simulink model "TideVCU"  (R2021b)
settings: Solver=FixedStepDiscrete  StartTime=0.0  StopTime=10.0  RelTol=1e-3
undefined symbols (not defined in the file): dataName, enumName, enumValue, GCM, raptor_get_safe_string
libraries: Raptor_lib x93, simulink x8
(part 2 of 3)

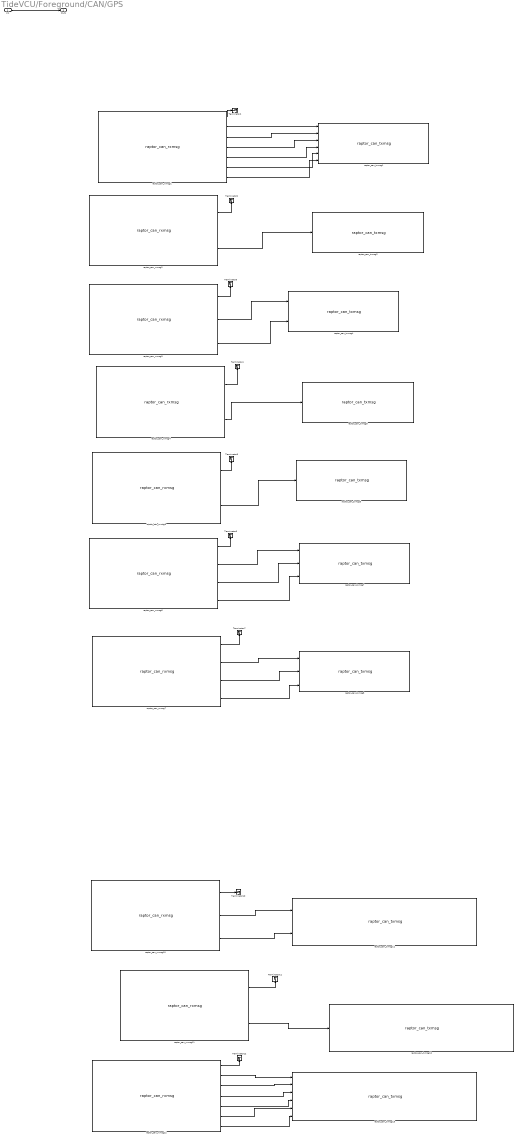
== system TideVCU/Foreground/CAN/GPS ==
  In1 : Inport
  Terminator{1..7,10..12} (10 alike) : Terminator
  raptor_can_rxmsg1 : Raptor_lib/CAN/raptor_can_rxmsg  canDefinition=struct('dbcFile', 'gps_out.dbc','message', 'accelxyz_temp_vertaxis_orientati','comment', '','signals', {{'accelx','accely','accelz','orientation','temp','vert_axis'}},'enabled', [ 1 1 1 1 1 1;],'scaled', [ 1 1 1 1 1 1;],'canBus', '''CAN1''','messageID', [ 1536;],'idMask', [ 536870911;],'payloadMask', [],'payloadValue', [],'period', [ 0;],'mailbox', '''''','queueSize', [ 1;],'label', [ 0;],'ver', [ 2;],'showID', [ 0;],'showRaw', [ 0;],'showRawMsg', [ 0;],'showAge', [ 1;],'fill', [ 0;],'editID', [ 0;],'signalOrder', [ 1;],'signalAscDes', [ 1;])  canBus='CAN1'  mailbox=''  payloadMask=[]  payloadValue=[]  idMask=hex2dec('1FFFFFFF')  queueSize=1  showID=0  label=0  fill=0  id=1536  showRaw=0  showAge=1  signalOrder=1  signalInfo={{struct('Name', 'accelx','Startbit', [ 0;],'SignalSize', [ 16;],'ByteOrder', 'LittleEndian','ValueType', 'SIGNED','Class', 'int16','Signed', [ 1;],'Factor', [ 3.91;],'Offset', [ 0;],'Min', [ 0;],'Max', [ 0;],'Units', '','Comment', '','StartBit', [ 0;]),struct('Name', 'accely','Startbit', [ 0;],'SignalSize', [ 16;],'ByteOrder', 'LittleEndian','ValueType', 'SIGNED','Class', 'int16','Signed', [ 1;],'Factor', [ 3.91;],'Offset', [ 0;],'Min', [ 0;],'Max', [ 0;],'Units', '','Comment', '','StartBit', [ 16;]),struct('Name', 'accelz','Startbit', [ 0;],'SignalSize', [ 16;],'ByteOrder', 'LittleEndian','ValueType', 'SIGNED','Class', 'int16','Signed', [ 1;],'Factor', [ 3.91;],'Offset', [ 0;],'Min', [ 0;],'Max', [ 0;],'Units', '','Comment', '','StartBit', [ 32;]),struct('Name', 'orientation','Startbit', [ 0;],'SignalSize', [ 3;],'ByteOrder', 'LittleEndian','ValueType', 'SIGNED','Class', 'int8','Signed', [ 1;],'Factor', [ 1;],'Offset', [ 0;],'Min', [ 0;],'Max', [ 0;],'Units', '','Comment', '','StartBit', [ 58;]),struct('Name', 'temp','Startbit', [ 0;],'SignalSize', [ 8;],'ByteOrder', 'LittleEndian','ValueType', 'SIGNED','Class', 'int8','Signed', [ 1;],'Factor', [ 0.5;],'Offset', [ 24;],'Min', [ 0;],'Max', [ 0;],'Units', 'c','Comment', '','StartBit', [ 48;]),struct('Name', 'vert_axis','Startbit', [ 0;],'SignalSize', [ 2;],'ByteOrder', 'LittleEndian','ValueType', 'SIGNED','Class', 'int8','Signed', [ 1;],'Factor', [ 1;],'Offset', [ 0;],'Min', [ 0;],'Max', [ 0;],'Units', '','Comment', '','StartBit', [ 56;])}}  showRawMsg=0
      settings: SourceProductName=Raptor
  raptor_can_rxmsg10 : Raptor_lib/CAN/raptor_can_rxmsg  canDefinition=struct('dbcFile', 'gps_out.dbc','message', 'rotation_xy','comment', '','signals', {{'rotationx','rotationy'}},'enabled', [ 1 1;],'scaled', [ 1 1;],'canBus', '''CAN2''','messageID', [ 1552;],'idMask', [ 536870911;],'payloadMask', [],'payloadValue', [],'period', [ 0;],'mailbox', '''''','queueSize', [ 1;],'label', [ 0;],'ver', [ 2;],'showID', [ 0;],'showRaw', [ 0;],'showRawMsg', [ 0;],'showAge', [ 1;],'fill', [ 0;],'editID', [ 0;],'signalOrder', [ 1;],'signalAscDes', [ 1;])  canBus='CAN2'  mailbox=''  payloadMask=[]  payloadValue=[]  idMask=hex2dec('1FFFFFFF')  queueSize=1  showID=0  label=0  fill=0  id=1552  showRaw=0  showAge=1  signalOrder=1  signalInfo={{struct('Name', 'rotationx','Startbit', [ 0;],'SignalSize', [ 32;],'ByteOrder', 'LittleEndian','ValueType', 'FLOAT32','Class', 'single','Signed', [ 1;],'Factor', [ 1;],'Offset', [ 0;],'Min', [ 0;],'Max', [ 0;],'Units', '','Comment', '','StartBit', [ 0;]),struct('Name', 'rotationy','Startbit', [ 0;],'SignalSize', [ 32;],'ByteOrder', 'LittleEndian','ValueType', 'FLOAT32','Class', 'single','Signed', [ 1;],'Factor', [ 1;],'Offset', [ 0;],'Min', [ 0;],'Max', [ 0;],'Units', '','Comment', '','StartBit', [ 32;])}}  showRawMsg=0
      settings: SourceProductName=Raptor
  raptor_can_rxmsg11 : Raptor_lib/CAN/raptor_can_rxmsg  canDefinition=struct('dbcFile', 'gps_out.dbc','message', 'rotationz','comment', '','signals', {{'rotationz'}},'enabled', [ 1;],'scaled', [ 1;],'canBus', '''CAN2''','messageID', [ 1553;],'idMask', [ 536870911;],'payloadMask', [],'payloadValue', [],'period', [ 0;],'mailbox', '''''','queueSize', [ 1;],'label', [ 0;],'ver', [ 2;],'showID', [ 0;],'showRaw', [ 0;],'showRawMsg', [ 0;],'showAge', [ 1;],'fill', [ 0;],'editID', [ 0;],'signalOrder', [ 1;],'signalAscDes', [ 1;])  canBus='CAN2'  mailbox=''  payloadMask=[]  payloadValue=[]  idMask=hex2dec('1FFFFFFF')  queueSize=1  showID=0  label=0  fill=0  id=1553  showRaw=0  showAge=1  signalOrder=1  signalInfo={{struct('Name', 'rotationz','Startbit', [ 0;],'SignalSize', [ 32;],'ByteOrder', 'LittleEndian','ValueType', 'FLOAT32','Class', 'single','Signed', [ 1;],'Factor', [ 1;],'Offset', [ 0;],'Min', [ 0;],'Max', [ 0;],'Units', '','Comment', '','StartBit', [ 0;])}}  showRawMsg=0
      settings: SourceProductName=Raptor
  raptor_can_rxmsg12 : Raptor_lib/CAN/raptor_can_rxmsg  canDefinition=struct('dbcFile', 'gps_out.dbc','message', 'IO','comment', '','signals', {{'Device_ID','Din1_status','Din2_status','Dout_status','GPS_powerStatus','SD_present'}},'enabled', [ 1 1 1 1 1 1;],'scaled', [ 1 1 1 1 1 1;],'canBus', '''CAN2''','messageID', [ 1584;],'idMask', [ 536870911;],'payloadMask', [],'payloadValue', [],'period', [ 0;],'mailbox', '''''','queueSize', [ 1;],'label', [ 0;],'ver', [ 2;],'showID', [ 0;],'showRaw', [ 0;],'showRawMsg', [ 0;],'showAge', [ 1;],'fill', [ 0;],'editID', [ 0;],'signalOrder', [ 1;],'signalAscDes', [ 1;])  canBus='CAN2'  mailbox=''  payloadMask=[]  payloadValue=[]  idMask=hex2dec('1FFFFFFF')  queueSize=1  showID=0  label=0  fill=0  id=1584  showRaw=0  showAge=1  signalOrder=1  signalInfo={{struct('Name', 'Din1_status','Startbit', [ 0;],'SignalSize', [ 1;],'ByteOrder', 'LittleEndian','ValueType', 'UNSIGNED','Class', 'uint8','Signed', [ 0;],'Factor', [ 1;],'Offset', [ 0;],'Min', [ 0;],'Max', [ 0;],'Units', '','Comment', '','StartBit', [ 0;]),struct('Name', 'Din2_status','Startbit', [ 0;],'SignalSize', [ 1;],'ByteOrder', 'LittleEndian','ValueType', 'UNSIGNED','Class', 'uint8','Signed', [ 0;],'Factor', [ 1;],'Offset', [ 0;],'Min', [ 0;],'Max', [ 0;],'Units', '','Comment', '','StartBit', [ 1;]),struct('Name', 'Dout_status','Startbit', [ 0;],'SignalSize', [ 1;],'ByteOrder', 'LittleEndian','ValueType', 'UNSIGNED','Class', 'uint8','Signed', [ 0;],'Factor', [ 1;],'Offset', [ 0;],'Min', [ 0;],'Max', [ 0;],'Units', '','Comment', '','StartBit', [ 2;]),struct('Name', 'SD_present','Startbit', [ 0;],'SignalSize', [ 1;],'ByteOrder', 'LittleEndian','ValueType', 'UNSIGNED','Class', 'uint8','Signed', [ 0;],'Factor', [ 1;],'Offset', [ 0;],'Min', [ 0;],'Max', [ 0;],'Units', '','Comment', '','StartBit', [ 3;]),struct('Name', 'GPS_powerStatus','Startbit', [ 0;],'SignalSize', [ 1;],'ByteOrder', 'LittleEndian','ValueType', 'UNSIGNED','Class', 'uint8','Signed', [ 0;],'Factor', [ 1;],'Offset', [ 0;],'Min', [ 0;],'Max', [ 0;],'Units', '','Comment', '','StartBit', [ 4;]),struct('Name', 'Device_ID','Startbit', [ 0;],'SignalSize', [ 3;],'ByteOrder', 'LittleEndian','ValueType', 'UNSIGNED','Class', 'uint8','Signed', [ 0;],'Factor', [ 1;],'Offset', [ 0;],'Min', [ 0;],'Max', [ 0;],'Units', '','Comment', '','StartBit', [ 5;])}}  showRawMsg=0
      settings: SourceProductName=Raptor
  raptor_can_rxmsg2 : Raptor_lib/CAN/raptor_can_rxmsg  canDefinition=struct('dbcFile', 'gps_out.dbc','message', 'gps_altitude','comment', '','signals', {{'altitude'}},'enabled', [ 1;],'scaled', [ 1;],'canBus', '''CAN1''','messageID', [ 1572;],'idMask', [ 536870911;],'payloadMask', [],'payloadValue', [],'period', [ 0;],'mailbox', '''''','queueSize', [ 1;],'label', [ 0;],'ver', [ 2;],'showID', [ 0;],'showRaw', [ 0;],'showRawMsg', [ 0;],'showAge', [ 1;],'fill', [ 0;],'editID', [ 0;],'signalOrder', [ 1;],'signalAscDes', [ 1;])  canBus='CAN1'  mailbox=''  payloadMask=[]  payloadValue=[]  idMask=hex2dec('1FFFFFFF')  queueSize=1  showID=0  label=0  fill=0  id=1572  showRaw=0  showAge=1  signalOrder=1  signalInfo={{struct('Name', 'altitude','Startbit', [ 0;],'SignalSize', [ 32;],'ByteOrder', 'LittleEndian','ValueType', 'FLOAT32','Class', 'single','Signed', [ 1;],'Factor', [ 1;],'Offset', [ 0;],'Min', [ 0;],'Max', [ 0;],'Units', '','Comment', '','StartBit', [ 0;])}}  showRawMsg=0
      settings: SourceProductName=Raptor
  raptor_can_rxmsg3 : Raptor_lib/CAN/raptor_can_rxmsg  canDefinition=struct('dbcFile', 'gps_out.dbc','message', 'gps_course_speed','comment', '','signals', {{'gps_course','gps_speed'}},'enabled', [ 1 1;],'scaled', [ 1 1;],'canBus', '''CAN2''','messageID', [ 1569;],'idMask', [ 536870911;],'payloadMask', [],'payloadValue', [],'period', [ 0;],'mailbox', '''''','queueSize', [ 1;],'label', [ 0;],'ver', [ 2;],'showID', [ 0;],'showRaw', [ 0;],'showRawMsg', [ 0;],'showAge', [ 1;],'fill', [ 0;],'editID', [ 0;],'signalOrder', [ 1;],'signalAscDes', [ 1;])  canBus='CAN2'  mailbox=''  payloadMask=[]  payloadValue=[]  idMask=hex2dec('1FFFFFFF')  queueSize=1  showID=0  label=0  fill=0  id=1569  showRaw=0  showAge=1  signalOrder=1  signalInfo={{struct('Name', 'gps_course','Startbit', [ 0;],'SignalSize', [ 32;],'ByteOrder', 'LittleEndian','ValueType', 'FLOAT32','Class', 'single','Signed', [ 1;],'Factor', [ 1;],'Offset', [ 0;],'Min', [ 0;],'Max', [ 0;],'Units', '','Comment', 'float, degrees','StartBit', [ 0;]),struct('Name', 'gps_speed','Startbit', [ 0;],'SignalSize', [ 32;],'ByteOrder', 'LittleEndian','ValueType', 'FLOAT32','Class', 'single','Signed', [ 1;],'Factor', [ 1;],'Offset', [ 0;],'Min', [ 0;],'Max', [ 0;],'Units', '','Comment', 'float, km/h','StartBit', [ 32;])}}  showRawMsg=0
      settings: SourceProductName=Raptor
  raptor_can_rxmsg4 : Raptor_lib/CAN/raptor_can_rxmsg  canDefinition=struct('dbcFile', 'gps_out.dbc','message', 'gps_delusionsA','comment', '','signals', {{'hdop','pdop'}},'enabled', [ 0 1;],'scaled', [ 1 1;],'canBus', '''CAN2''','messageID', [ 1573;],'idMask', [ 536870911;],'payloadMask', [],'payloadValue', [],'period', [ 0;],'mailbox', '''''','queueSize', [ 1;],'label', [ 0;],'ver', [ 2;],'showID', [ 0;],'showRaw', [ 0;],'showRawMsg', [ 0;],'showAge', [ 1;],'fill', [ 0;],'editID', [ 0;],'signalOrder', [ 1;],'signalAscDes', [ 1;])  canBus='CAN2'  mailbox=''  payloadMask=[]  payloadValue=[]  idMask=hex2dec('1FFFFFFF')  queueSize=1  showID=0  label=0  fill=0  id=1573  showRaw=0  showAge=1  signalOrder=1  signalInfo={{struct('Name', 'hdop','Startbit', [ 0;],'SignalSize', [ 32;],'ByteOrder', 'LittleEndian','ValueType', 'FLOAT32','Class', 'single','Signed', [ 1;],'Factor', [ 1;],'Offset', [ 0;],'Min', [ 0;],'Max', [ 0;],'Units', '','Comment', 'lower=better','StartBit', [ 32;]),struct('Name', 'pdop','Startbit', [ 0;],'SignalSize', [ 32;],'ByteOrder', 'LittleEndian','ValueType', 'FLOAT32','Class', 'single','Signed', [ 1;],'Factor', [ 1;],'Offset', [ 0;],'Min', [ 0;],'Max', [ 0;],'Units', '','Comment', 'lower=better','StartBit', [ 0;])}}  showRawMsg=0
      settings: SourceProductName=Raptor
  raptor_can_rxmsg5 : Raptor_lib/CAN/raptor_can_rxmsg  canDefinition=struct('dbcFile', 'gps_out.dbc','message', 'gps_delusionsB','comment', '','signals', {{'vdop'}},'enabled', [ 1;],'scaled', [ 1;],'canBus', '''CAN2''','messageID', [ 1574;],'idMask', [ 536870911;],'payloadMask', [],'payloadValue', [],'period', [ 0;],'mailbox', '''''','queueSize', [ 1;],'label', [ 0;],'ver', [ 2;],'showID', [ 0;],'showRaw', [ 0;],'showRawMsg', [ 0;],'showAge', [ 1;],'fill', [ 0;],'editID', [ 0;],'signalOrder', [ 1;],'signalAscDes', [ 1;])  canBus='CAN2'  mailbox=''  payloadMask=[]  payloadValue=[]  idMask=hex2dec('1FFFFFFF')  queueSize=1  showID=0  label=0  fill=0  id=1574  showRaw=0  showAge=1  signalOrder=1  signalInfo={{struct('Name', 'vdop','Startbit', [ 0;],'SignalSize', [ 32;],'ByteOrder', 'LittleEndian','ValueType', 'FLOAT32','Class', 'single','Signed', [ 1;],'Factor', [ 1;],'Offset', [ 0;],'Min', [ 0;],'Max', [ 0;],'Units', '','Comment', 'lower=better','StartBit', [ 0;])}}  showRawMsg=0
      settings: SourceProductName=Raptor
  raptor_can_rxmsg6 : Raptor_lib/CAN/raptor_can_rxmsg  canDefinition=struct('dbcFile', 'gps_out.dbc','message', 'gps_latitude','comment', '','signals', {{'indicator_north_south','latitude_degrees','latitude_minutes'}},'enabled', [ 1 1 1;],'scaled', [ 1 1 1;],'canBus', '''CAN2''','messageID', [ 1571;],'idMask', [ 536870911;],'payloadMask', [],'payloadValue', [],'period', [ 0;],'mailbox', '''''','queueSize', [ 1;],'label', [ 0;],'ver', [ 2;],'showID', [ 0;],'showRaw', [ 0;],'showRawMsg', [ 0;],'showAge', [ 1;],'fill', [ 0;],'editID', [ 0;],'signalOrder', [ 1;],'signalAscDes', [ 1;])  canBus='CAN2'  mailbox=''  payloadMask=[]  payloadValue=[]  idMask=hex2dec('1FFFFFFF')  queueSize=1  showID=0  label=0  fill=0  id=1571  showRaw=0  showAge=1  signalOrder=1  signalInfo={{struct('Name', 'latitude_minutes','Startbit', [ 0;],'SignalSize', [ 32;],'ByteOrder', 'LittleEndian','ValueType', 'FLOAT32','Class', 'single','Signed', [ 1;],'Factor', [ 1;],'Offset', [ 0;],'Min', [ 0;],'Max', [ 0;],'Units', '','Comment', 'float','StartBit', [ 0;]),struct('Name', 'latitude_degrees','Startbit', [ 0;],'SignalSize', [ 16;],'ByteOrder', 'LittleEndian','ValueType', 'SIGNED','Class', 'int16','Signed', [ 1;],'Factor', [ 1;],'Offset', [ 0;],'Min', [ 0;],'Max', [ 0;],'Units', '','Comment', '','StartBit', [ 32;]),struct('Name', 'indicator_north_south','Startbit', [ 0;],'SignalSize', [ 8;],'ByteOrder', 'LittleEndian','ValueType', 'SIGNED','Class', 'int8','Signed', [ 1;],'Factor', [ 1;],'Offset', [ 0;],'Min', [ 0;],'Max', [ 0;],'Units', '','Comment', '0=init','StartBit', [ 48;])}}  showRawMsg=0
      settings: SourceProductName=Raptor
  raptor_can_rxmsg7 : Raptor_lib/CAN/raptor_can_rxmsg  canDefinition=struct('dbcFile', 'gps_out.dbc','message', 'gps_longitude','comment', '','signals', {{'indicator_East_West','longitude_degrees','longitude_minutes'}},'enabled', [ 1 1 1;],'scaled', [ 1 1 1;],'canBus', '''CAN2''','messageID', [ 1570;],'idMask', [ 536870911;],'payloadMask', [],'payloadValue', [],'period', [ 0;],'mailbox', '''''','queueSize', [ 1;],'label', [ 0;],'ver', [ 2;],'showID', [ 0;],'showRaw', [ 0;],'showRawMsg', [ 0;],'showAge', [ 1;],'fill', [ 0;],'editID', [ 0;],'signalOrder', [ 1;],'signalAscDes', [ 1;])  canBus='CAN2'  mailbox=''  payloadMask=[]  payloadValue=[]  idMask=hex2dec('1FFFFFFF')  queueSize=1  showID=0  label=0  fill=0  id=1570  showRaw=0  showAge=1  signalOrder=1  signalInfo={{struct('Name', 'longitude_minutes','Startbit', [ 0;],'SignalSize', [ 32;],'ByteOrder', 'LittleEndian','ValueType', 'FLOAT32','Class', 'single','Signed', [ 1;],'Factor', [ 1;],'Offset', [ 0;],'Min', [ 0;],'Max', [ 0;],'Units', '','Comment', 'float','StartBit', [ 0;]),struct('Name', 'longitude_degrees','Startbit', [ 0;],'SignalSize', [ 16;],'ByteOrder', 'LittleEndian','ValueType', 'SIGNED','Class', 'int16','Signed', [ 1;],'Factor', [ 1;],'Offset', [ 0;],'Min', [ 0;],'Max', [ 0;],'Units', '','Comment', '','StartBit', [ 32;]),struct('Name', 'indicator_East_West','Startbit', [ 0;],'SignalSize', [ 8;],'ByteOrder', 'LittleEndian','ValueType', 'UNSIGNED','Class', 'uint8','Signed', [ 0;],'Factor', [ 1;],'Offset', [ 0;],'Min', [ 0;],'Max', [ 0;],'Units', '','Comment', '0=init','StartBit', [ 48;])}}  showRawMsg=0
      settings: SourceProductName=Raptor
  raptor_can_txmsg1 : Raptor_lib/CAN/raptor_can_txmsg  canDefinition=struct('dbcFile', 'gps_out.dbc','message', 'accelxyz_temp_vertaxis_orientati','comment', '','signals', {{'accelx','accely','accelz','orientation','temp','vert_axis'}},'enabled', [ 1 1 1 1 1 1;],'scaled', [ 1 1 1 1 1 1;],'canBus', '''CAN1''','messageID', [ 1536;],'idMask', [ 536870911;],'payloadMask', [],'payloadValue', [],'period', [ 0;],'mailbox', '','queueSize', [ 1;],'label', [ 0;],'ver', [ 2;],'showID', [ 0;],'showRaw', [ 0;],'showRawMsg', [ 0;],'fill', [ 0;],'editID', [ 0;],'signalOrder', [ 1;],'signalAscDes', [ 1;])  canBus='CAN1'  queueSize=1  payloadMask=[]  payloadValue=[]  period=0  showID=0  label=0  idMask=hex2dec('1FFFFFFF')  fill=0  id=1536  showRaw=0  signalOrder=1  signalInfo={{struct('Name', 'accelx','Startbit', [ 0;],'SignalSize', [ 16;],'ByteOrder', 'LittleEndian','ValueType', 'SIGNED','Class', 'int16','Signed', [ 1;],'Factor', [ 3.91;],'Offset', [ 0;],'Min', [ 0;],'Max', [ 0;],'Units', '','Comment', '','StartBit', [ 0;]),struct('Name', 'accely','Startbit', [ 0;],'SignalSize', [ 16;],'ByteOrder', 'LittleEndian','ValueType', 'SIGNED','Class', 'int16','Signed', [ 1;],'Factor', [ 3.91;],'Offset', [ 0;],'Min', [ 0;],'Max', [ 0;],'Units', '','Comment', '','StartBit', [ 16;]),struct('Name', 'accelz','Startbit', [ 0;],'SignalSize', [ 16;],'ByteOrder', 'LittleEndian','ValueType', 'SIGNED','Class', 'int16','Signed', [ 1;],'Factor', [ 3.91;],'Offset', [ 0;],'Min', [ 0;],'Max', [ 0;],'Units', '','Comment', '','StartBit', [ 32;]),struct('Name', 'temp','Startbit', [ 0;],'SignalSize', [ 8;],'ByteOrder', 'LittleEndian','ValueType', 'SIGNED','Class', 'int8','Signed', [ 1;],'Factor', [ 0.5;],'Offset', [ 24;],'Min', [ 0;],'Max', [ 0;],'Units', 'c','Comment', '','StartBit', [ 48;]),struct('Name', 'vert_axis','Startbit', [ 0;],'SignalSize', [ 2;],'ByteOrder', 'LittleEndian','ValueType', 'SIGNED','Class', 'int8','Signed', [ 1;],'Factor', [ 1;],'Offset', [ 0;],'Min', [ 0;],'Max', [ 0;],'Units', '','Comment', '','StartBit', [ 56;]),struct('Name', 'orientation','Startbit', [ 0;],'SignalSize', [ 3;],'ByteOrder', 'LittleEndian','ValueType', 'SIGNED','Class', 'int8','Signed', [ 1;],'Factor', [ 1;],'Offset', [ 0;],'Min', [ 0;],'Max', [ 0;],'Units', '','Comment', '','StartBit', [ 58;])}}
      settings: SourceProductName=Raptor
  raptor_can_txmsg11 : Raptor_lib/CAN/raptor_can_txmsg  canDefinition=struct('dbcFile', 'gps_out.dbc','message', 'rotation_xy','comment', '','signals', {{'rotationx','rotationy'}},'enabled', [ 1 1;],'scaled', [ 1 1;],'canBus', '''CAN1''','messageID', [ 1552;],'idMask', [ 536870911;],'payloadMask', [],'payloadValue', [],'period', [ 0;],'mailbox', '','queueSize', [ 1;],'label', [ 0;],'ver', [ 2;],'showID', [ 0;],'showRaw', [ 0;],'showRawMsg', [ 0;],'fill', [ 0;],'editID', [ 0;],'signalOrder', [ 1;],'signalAscDes', [ 1;])  canBus='CAN1'  queueSize=1  payloadMask=[]  payloadValue=[]  period=0  showID=0  label=0  idMask=hex2dec('1FFFFFFF')  fill=0  id=1552  showRaw=0  signalOrder=1  signalInfo={{struct('Name', 'rotationx','Startbit', [ 0;],'SignalSize', [ 32;],'ByteOrder', 'LittleEndian','ValueType', 'FLOAT32','Class', 'single','Signed', [ 1;],'Factor', [ 1;],'Offset', [ 0;],'Min', [ 0;],'Max', [ 0;],'Units', '','Comment', '','StartBit', [ 0;]),struct('Name', 'rotationy','Startbit', [ 0;],'SignalSize', [ 32;],'ByteOrder', 'LittleEndian','ValueType', 'FLOAT32','Class', 'single','Signed', [ 1;],'Factor', [ 1;],'Offset', [ 0;],'Min', [ 0;],'Max', [ 0;],'Units', '','Comment', '','StartBit', [ 32;])}}
      settings: SourceProductName=Raptor
  raptor_can_txmsg12 : Raptor_lib/CAN/raptor_can_txmsg  canDefinition=struct('dbcFile', 'gps_out.dbc','message', 'rotationz','comment', '','signals', {{'rotationz'}},'enabled', [ 1;],'scaled', [ 1;],'canBus', '''CAN1''','messageID', [ 1553;],'idMask', [ 536870911;],'payloadMask', [],'payloadValue', [],'period', [ 0;],'mailbox', '','queueSize', [ 1;],'label', [ 0;],'ver', [ 2;],'showID', [ 0;],'showRaw', [ 0;],'showRawMsg', [ 0;],'fill', [ 0;],'editID', [ 0;],'signalOrder', [ 1;],'signalAscDes', [ 1;])  canBus='CAN1'  queueSize=1  payloadMask=[]  payloadValue=[]  period=0  showID=0  label=0  idMask=hex2dec('1FFFFFFF')  fill=0  id=1553  showRaw=0  signalOrder=1  signalInfo={{struct('Name', 'rotationz','Startbit', [ 0;],'SignalSize', [ 32;],'ByteOrder', 'LittleEndian','ValueType', 'FLOAT32','Class', 'single','Signed', [ 1;],'Factor', [ 1;],'Offset', [ 0;],'Min', [ 0;],'Max', [ 0;],'Units', '','Comment', '','StartBit', [ 0;])}}
      settings: SourceProductName=Raptor
  raptor_can_txmsg13 : Raptor_lib/CAN/raptor_can_txmsg  canDefinition=struct('dbcFile', 'gps_out.dbc','message', 'IO','comment', '','signals', {{'Device_ID','Din1_status','Din2_status','Dout_status','GPS_powerStatus','SD_present'}},'enabled', [ 1 1 1 1 1 1;],'scaled', [ 1 1 1 1 1 1;],'canBus', '''CAN1''','messageID', [ 1584;],'idMask', [ 536870911;],'payloadMask', [],'payloadValue', [],'period', [ 0;],'mailbox', '','queueSize', [ 1;],'label', [ 0;],'ver', [ 2;],'showID', [ 0;],'showRaw', [ 0;],'showRawMsg', [ 0;],'fill', [ 0;],'editID', [ 0;],'signalOrder', [ 1;],'signalAscDes', [ 1;])  canBus='CAN1'  queueSize=1  payloadMask=[]  payloadValue=[]  period=0  showID=0  label=0  idMask=hex2dec('1FFFFFFF')  fill=0  id=1584  showRaw=0  signalOrder=1  signalInfo={{struct('Name', 'Din1_status','Startbit', [ 0;],'SignalSize', [ 1;],'ByteOrder', 'LittleEndian','ValueType', 'UNSIGNED','Class', 'uint8','Signed', [ 0;],'Factor', [ 1;],'Offset', [ 0;],'Min', [ 0;],'Max', [ 0;],'Units', '','Comment', '','StartBit', [ 0;]),struct('Name', 'Din2_status','Startbit', [ 0;],'SignalSize', [ 1;],'ByteOrder', 'LittleEndian','ValueType', 'UNSIGNED','Class', 'uint8','Signed', [ 0;],'Factor', [ 1;],'Offset', [ 0;],'Min', [ 0;],'Max', [ 0;],'Units', '','Comment', '','StartBit', [ 1;]),struct('Name', 'Dout_status','Startbit', [ 0;],'SignalSize', [ 1;],'ByteOrder', 'LittleEndian','ValueType', 'UNSIGNED','Class', 'uint8','Signed', [ 0;],'Factor', [ 1;],'Offset', [ 0;],'Min', [ 0;],'Max', [ 0;],'Units', '','Comment', '','StartBit', [ 2;]),struct('Name', 'SD_present','Startbit', [ 0;],'SignalSize', [ 1;],'ByteOrder', 'LittleEndian','ValueType', 'UNSIGNED','Class', 'uint8','Signed', [ 0;],'Factor', [ 1;],'Offset', [ 0;],'Min', [ 0;],'Max', [ 0;],'Units', '','Comment', '','StartBit', [ 3;]),struct('Name', 'GPS_powerStatus','Startbit', [ 0;],'SignalSize', [ 1;],'ByteOrder', 'LittleEndian','ValueType', 'UNSIGNED','Class', 'uint8','Signed', [ 0;],'Factor', [ 1;],'Offset', [ 0;],'Min', [ 0;],'Max', [ 0;],'Units', '','Comment', '','StartBit', [ 4;]),struct('Name', 'Device_ID','Startbit', [ 0;],'SignalSize', [ 3;],'ByteOrder', 'LittleEndian','ValueType', 'UNSIGNED','Class', 'uint8','Signed', [ 0;],'Factor', [ 1;],'Offset', [ 0;],'Min', [ 0;],'Max', [ 0;],'Units', '','Comment', '','StartBit', [ 5;])}}
      settings: SourceProductName=Raptor
  raptor_can_txmsg2 : Raptor_lib/CAN/raptor_can_txmsg  canDefinition=struct('dbcFile', 'gps_out.dbc','message', 'gps_altitude','comment', '','signals', {{'altitude'}},'enabled', [ 1;],'scaled', [ 1;],'canBus', '''CAN1''','messageID', [ 1572;],'idMask', [ 536870911;],'payloadMask', [],'payloadValue', [],'period', [ 0;],'mailbox', '','queueSize', [ 1;],'label', [ 0;],'ver', [ 2;],'showID', [ 0;],'showRaw', [ 0;],'showRawMsg', [ 0;],'fill', [ 0;],'editID', [ 0;],'signalOrder', [ 1;],'signalAscDes', [ 1;])  canBus='CAN1'  queueSize=1  payloadMask=[]  payloadValue=[]  period=0  showID=0  label=0  idMask=hex2dec('1FFFFFFF')  fill=0  id=1572  showRaw=0  signalOrder=1  signalInfo={{struct('Name', 'altitude','Startbit', [ 0;],'SignalSize', [ 32;],'ByteOrder', 'LittleEndian','ValueType', 'FLOAT32','Class', 'single','Signed', [ 1;],'Factor', [ 1;],'Offset', [ 0;],'Min', [ 0;],'Max', [ 0;],'Units', '','Comment', '','StartBit', [ 0;])}}
      settings: SourceProductName=Raptor
  raptor_can_txmsg4 : Raptor_lib/CAN/raptor_can_txmsg  canDefinition=struct('dbcFile', 'gps_out.dbc','message', 'gps_course_speed','comment', '','signals', {{'gps_course','gps_speed'}},'enabled', [ 1 1;],'scaled', [ 1 1;],'canBus', '''CAN1''','messageID', [ 1569;],'idMask', [ 536870911;],'payloadMask', [],'payloadValue', [],'period', [ 0;],'mailbox', '','queueSize', [ 1;],'label', [ 0;],'ver', [ 2;],'showID', [ 0;],'showRaw', [ 0;],'showRawMsg', [ 0;],'fill', [ 0;],'editID', [ 0;],'signalOrder', [ 1;],'signalAscDes', [ 1;])  canBus='CAN1'  queueSize=1  payloadMask=[]  payloadValue=[]  period=0  showID=0  label=0  idMask=hex2dec('1FFFFFFF')  fill=0  id=1569  showRaw=0  signalOrder=1  signalInfo={{struct('Name', 'gps_course','Startbit', [ 0;],'SignalSize', [ 32;],'ByteOrder', 'LittleEndian','ValueType', 'FLOAT32','Class', 'single','Signed', [ 1;],'Factor', [ 1;],'Offset', [ 0;],'Min', [ 0;],'Max', [ 0;],'Units', '','Comment', 'float, degrees','StartBit', [ 0;]),struct('Name', 'gps_speed','Startbit', [ 0;],'SignalSize', [ 32;],'ByteOrder', 'LittleEndian','ValueType', 'FLOAT32','Class', 'single','Signed', [ 1;],'Factor', [ 1;],'Offset', [ 0;],'Min', [ 0;],'Max', [ 0;],'Units', '','Comment', 'float, km/h','StartBit', [ 32;])}}
      settings: SourceProductName=Raptor
  raptor_can_txmsg5 : Raptor_lib/CAN/raptor_can_txmsg  canDefinition=struct('dbcFile', 'gps_out.dbc','message', 'gps_delusionsA','comment', '','signals', {{'hdop','pdop'}},'enabled', [ 0 1;],'scaled', [ 1 1;],'canBus', '''CAN1''','messageID', [ 1573;],'idMask', [ 536870911;],'payloadMask', [],'payloadValue', [],'period', [ 0;],'mailbox', '','queueSize', [ 1;],'label', [ 0;],'ver', [ 2;],'showID', [ 0;],'showRaw', [ 0;],'showRawMsg', [ 0;],'fill', [ 0;],'editID', [ 0;],'signalOrder', [ 1;],'signalAscDes', [ 1;])  canBus='CAN1'  queueSize=1  payloadMask=[]  payloadValue=[]  period=0  showID=0  label=0  idMask=hex2dec('1FFFFFFF')  fill=0  id=1573  showRaw=0  signalOrder=1  signalInfo={{struct('Name', 'hdop','Startbit', [ 0;],'SignalSize', [ 32;],'ByteOrder', 'LittleEndian','ValueType', 'FLOAT32','Class', 'single','Signed', [ 1;],'Factor', [ 1;],'Offset', [ 0;],'Min', [ 0;],'Max', [ 0;],'Units', '','Comment', 'lower=better','StartBit', [ 32;]),struct('Name', 'pdop','Startbit', [ 0;],'SignalSize', [ 32;],'ByteOrder', 'LittleEndian','ValueType', 'FLOAT32','Class', 'single','Signed', [ 1;],'Factor', [ 1;],'Offset', [ 0;],'Min', [ 0;],'Max', [ 0;],'Units', '','Comment', 'lower=better','StartBit', [ 0;])}}
      settings: SourceProductName=Raptor
  raptor_can_txmsg6 : Raptor_lib/CAN/raptor_can_txmsg  canDefinition=struct('dbcFile', 'gps_out.dbc','message', 'gps_delusionsB','comment', '','signals', {{'vdop'}},'enabled', [ 1;],'scaled', [ 1;],'canBus', '''CAN1''','messageID', [ 1574;],'idMask', [ 536870911;],'payloadMask', [],'payloadValue', [],'period', [ 0;],'mailbox', '','queueSize', [ 1;],'label', [ 0;],'ver', [ 2;],'showID', [ 0;],'showRaw', [ 0;],'showRawMsg', [ 0;],'fill', [ 0;],'editID', [ 0;],'signalOrder', [ 1;],'signalAscDes', [ 1;])  canBus='CAN1'  queueSize=1  payloadMask=[]  payloadValue=[]  period=0  showID=0  label=0  idMask=hex2dec('1FFFFFFF')  fill=0  id=1574  showRaw=0  signalOrder=1  signalInfo={{struct('Name', 'vdop','Startbit', [ 0;],'SignalSize', [ 32;],'ByteOrder', 'LittleEndian','ValueType', 'FLOAT32','Class', 'single','Signed', [ 1;],'Factor', [ 1;],'Offset', [ 0;],'Min', [ 0;],'Max', [ 0;],'Units', '','Comment', 'lower=better','StartBit', [ 0;])}}
      settings: SourceProductName=Raptor
  raptor_can_txmsg7 : Raptor_lib/CAN/raptor_can_txmsg  canDefinition=struct('dbcFile', 'gps_out.dbc','message', 'gps_latitude','comment', '','signals', {{'indicator_north_south','latitude_degrees','latitude_minutes'}},'enabled', [ 1 1 1;],'scaled', [ 1 1 1;],'canBus', '''CAN1''','messageID', [ 1571;],'idMask', [ 536870911;],'payloadMask', [],'payloadValue', [],'period', [ 0;],'mailbox', '','queueSize', [ 1;],'label', [ 0;],'ver', [ 2;],'showID', [ 0;],'showRaw', [ 0;],'showRawMsg', [ 0;],'fill', [ 0;],'editID', [ 0;],'signalOrder', [ 1;],'signalAscDes', [ 1;])  canBus='CAN1'  queueSize=1  payloadMask=[]  payloadValue=[]  period=0  showID=0  label=0  idMask=hex2dec('1FFFFFFF')  fill=0  id=1571  showRaw=0  signalOrder=1  signalInfo={{struct('Name', 'latitude_minutes','Startbit', [ 0;],'SignalSize', [ 32;],'ByteOrder', 'LittleEndian','ValueType', 'FLOAT32','Class', 'single','Signed', [ 1;],'Factor', [ 1;],'Offset', [ 0;],'Min', [ 0;],'Max', [ 0;],'Units', '','Comment', 'float','StartBit', [ 0;]),struct('Name', 'latitude_degrees','Startbit', [ 0;],'SignalSize', [ 16;],'ByteOrder', 'LittleEndian','ValueType', 'SIGNED','Class', 'int16','Signed', [ 1;],'Factor', [ 1;],'Offset', [ 0;],'Min', [ 0;],'Max', [ 0;],'Units', '','Comment', '','StartBit', [ 32;]),struct('Name', 'indicator_north_south','Startbit', [ 0;],'SignalSize', [ 8;],'ByteOrder', 'LittleEndian','ValueType', 'SIGNED','Class', 'int8','Signed', [ 1;],'Factor', [ 1;],'Offset', [ 0;],'Min', [ 0;],'Max', [ 0;],'Units', '','Comment', '0=init','StartBit', [ 48;])}}
      settings: SourceProductName=Raptor
  raptor_can_txmsg8 : Raptor_lib/CAN/raptor_can_txmsg  canDefinition=struct('dbcFile', 'gps_out.dbc','message', 'gps_longitude','comment', '','signals', {{'indicator_East_West','longitude_degrees','longitude_minutes'}},'enabled', [ 1 1 1;],'scaled', [ 1 1 1;],'canBus', '''CAN1''','messageID', [ 1570;],'idMask', [ 536870911;],'payloadMask', [],'payloadValue', [],'period', [ 0;],'mailbox', '','queueSize', [ 1;],'label', [ 0;],'ver', [ 2;],'showID', [ 0;],'showRaw', [ 0;],'showRawMsg', [ 0;],'fill', [ 0;],'editID', [ 0;],'signalOrder', [ 1;],'signalAscDes', [ 1;])  canBus='CAN1'  queueSize=1  payloadMask=[]  payloadValue=[]  period=0  showID=0  label=0  idMask=hex2dec('1FFFFFFF')  fill=0  id=1570  showRaw=0  signalOrder=1  signalInfo={{struct('Name', 'longitude_minutes','Startbit', [ 0;],'SignalSize', [ 32;],'ByteOrder', 'LittleEndian','ValueType', 'FLOAT32','Class', 'single','Signed', [ 1;],'Factor', [ 1;],'Offset', [ 0;],'Min', [ 0;],'Max', [ 0;],'Units', '','Comment', 'float','StartBit', [ 0;]),struct('Name', 'longitude_degrees','Startbit', [ 0;],'SignalSize', [ 16;],'ByteOrder', 'LittleEndian','ValueType', 'SIGNED','Class', 'int16','Signed', [ 1;],'Factor', [ 1;],'Offset', [ 0;],'Min', [ 0;],'Max', [ 0;],'Units', '','Comment', '','StartBit', [ 32;]),struct('Name', 'indicator_East_West','Startbit', [ 0;],'SignalSize', [ 8;],'ByteOrder', 'LittleEndian','ValueType', 'UNSIGNED','Class', 'uint8','Signed', [ 0;],'Factor', [ 1;],'Offset', [ 0;],'Min', [ 0;],'Max', [ 0;],'Units', '','Comment', '0=init','StartBit', [ 48;])}}
      settings: SourceProductName=Raptor
  Out1 : Outport
  wires:
  In1/1 -> Out1/1
  raptor_can_rxmsg5/2 -> raptor_can_txmsg6/1
  raptor_can_rxmsg3/1 -> Terminator3/1
  raptor_can_rxmsg12/7 -> raptor_can_txmsg13/6
  raptor_can_rxmsg10/2 -> raptor_can_txmsg11/1
  raptor_can_rxmsg1/1 -> Terminator1/1
  raptor_can_rxmsg4/1 -> Terminator4/1
  raptor_can_rxmsg3/3 -> raptor_can_txmsg4/2
  raptor_can_rxmsg12/2 -> raptor_can_txmsg13/1
  raptor_can_rxmsg11/2 -> raptor_can_txmsg12/1
  raptor_can_rxmsg12/4 -> raptor_can_txmsg13/3
  raptor_can_rxmsg12/6 -> raptor_can_txmsg13/5
  raptor_can_rxmsg12/3 -> raptor_can_txmsg13/2
  raptor_can_rxmsg12/5 -> raptor_can_txmsg13/4
  raptor_can_rxmsg11/1 -> Terminator11/1
  raptor_can_rxmsg1/4 -> raptor_can_txmsg1/3
  raptor_can_rxmsg1/6 -> raptor_can_txmsg1/5
  raptor_can_rxmsg7/4 -> raptor_can_txmsg8/3
  raptor_can_rxmsg12/1 -> Terminator12/1
  raptor_can_rxmsg10/1 -> Terminator10/1
  raptor_can_rxmsg10/3 -> raptor_can_txmsg11/2
  raptor_can_rxmsg3/2 -> raptor_can_txmsg4/1
  raptor_can_rxmsg5/1 -> Terminator5/1
  raptor_can_rxmsg7/1 -> Terminator7/1
  raptor_can_rxmsg6/4 -> raptor_can_txmsg7/3
  raptor_can_rxmsg6/2 -> raptor_can_txmsg7/1
  raptor_can_rxmsg7/3 -> raptor_can_txmsg8/2
  raptor_can_rxmsg6/3 -> raptor_can_txmsg7/2
  raptor_can_rxmsg4/2 -> raptor_can_txmsg5/1
  raptor_can_rxmsg1/7 -> raptor_can_txmsg1/6
  raptor_can_rxmsg2/1 -> Terminator2/1
  raptor_can_rxmsg1/3 -> raptor_can_txmsg1/2
  raptor_can_rxmsg1/5 -> raptor_can_txmsg1/4
  raptor_can_rxmsg6/1 -> Terminator6/1
  raptor_can_rxmsg2/2 -> raptor_can_txmsg2/1
  raptor_can_rxmsg1/2 -> raptor_can_txmsg1/1
  raptor_can_rxmsg7/2 -> raptor_can_txmsg8/1

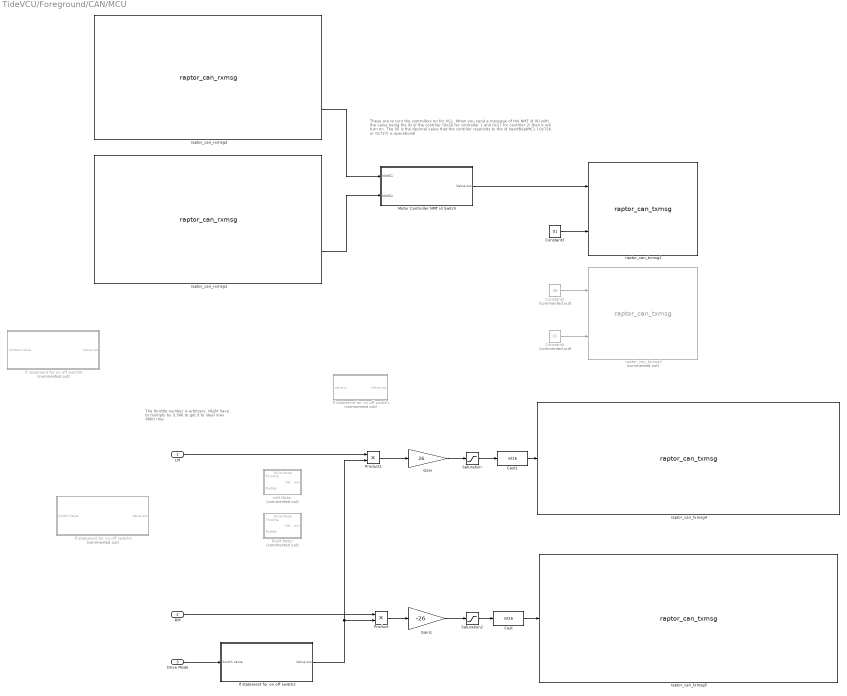
== system TideVCU/Foreground/CAN/MCU ==
  note: These are to turn the controllers on for VCL. When you send a message of the NMT id (0) with the value being the ID of the contrller (0x26 for controller 1 and 0x27 for contrller 2) then it will turn on. The 05 is the decimal value that the contrller responds to the id heartBeatMC1 ( 0x726 or 0x727) is operational
  note: The throttle number is arbitrary. Might have to multiply by 3.366 to get it to ideal max 4800 rmp
  LM : Inport
  RM : Inport  Port=2
  Drive Mode : Inport  Port=3
  Cast : DataTypeConversion  OutDataTypeStr=int16
  Cast1 : DataTypeConversion  OutDataTypeStr=int16
  Constant2 : Constant  Commented=on  Value=39
  Constant3 : Constant  Value=01
  Constant4 : Constant  Commented=on  Value=01
  Gain : Gain  Gain=26
  Gain1 : Gain  Gain=-26
  If statement for on off switch1 : Subsystem  Commented=on
  If statement for on off switch2 : Subsystem
  If statement for on off switch3 : Subsystem  Commented=on
  If statement for on off switch5 : Subsystem  Commented=on
  Left Motor : Subsystem  Commented=on
      settings: PortSchema="{\"entries\":[{\"content\":{\"sides\":[{\"content\":{\"connectorIds\":[\"In1\",\"In2\"]},\"type\":\"ConnectorPlacement.EquallySpacedRectSide\",\"uuid\":\"2083280e-5025-4497-a6f4-d95150e30dec\"},{\"content\":{\"connectorIds\":[\"Out1\"],\"side\":\"RIGHT\"},\"type\":\"ConnectorPlacement.EquallySpacedRectSide\",\"uuid\":\"61c851a0-d108-4419-a7df-f59beb96b75c\"},{\"content\":{\"connectorIds\":[\"In3\"],\"side\":\"TOP\"},\"type\":\"ConnectorPlacement.EquallySpacedRectSide\",\"uuid\":\"d9cef341-ca3e-4785-954e-89a8b6a8f97d\"}]},\"type\":\"ConnectorPlacement.EquallySpacedConnector\",\"uuid\":\"5877ad35-291b-4063-ae6a-1f18cb91c1ea\"}],\"packageUris\":[\"http://schema.mathworks.com/mf0/Connector/R2020b\"],\"version\":\"1.0\"}"
  Motor Controller NMT id Switch : Subsystem
  Product : Product
  Product1 : Product
  Right Motor : Subsystem  Commented=on
      settings: PortSchema="{\"entries\":[{\"content\":{\"sides\":[{\"content\":{\"connectorIds\":[\"In1\",\"In2\"]},\"type\":\"ConnectorPlacement.EquallySpacedRectSide\",\"uuid\":\"2083280e-5025-4497-a6f4-d95150e30dec\"},{\"content\":{\"connectorIds\":[\"Out1\"],\"side\":\"RIGHT\"},\"type\":\"ConnectorPlacement.EquallySpacedRectSide\",\"uuid\":\"61c851a0-d108-4419-a7df-f59beb96b75c\"},{\"content\":{\"connectorIds\":[\"In3\"],\"side\":\"TOP\"},\"type\":\"ConnectorPlacement.EquallySpacedRectSide\",\"uuid\":\"d9cef341-ca3e-4785-954e-89a8b6a8f97d\"}]},\"type\":\"ConnectorPlacement.EquallySpacedConnector\",\"uuid\":\"5877ad35-291b-4063-ae6a-1f18cb91c1ea\"}],\"packageUris\":[\"http://schema.mathworks.com/mf0/Connector/R2020b\"],\"version\":\"1.0\"}"
  Saturation : Saturate  UpperLimit=32767  LowerLimit=-32768
  Saturation2 : Saturate  UpperLimit=32767  LowerLimit=-32768
  raptor_can_rxmsg1 : Raptor_lib/CAN/raptor_can_rxmsg  canDefinition=struct('dbcFile', 'A1_MICH_EV_BOAT.dbc','message', 'heartBeatMC2','comment', '','signals', {{'hbMC2'}},'enabled', [ 1;],'scaled', [ 1;],'canBus', '''CAN3''','messageID', [ 1831;],'idMask', [ 536870911;],'payloadMask', [],'payloadValue', [],'period', [ 0;],'mailbox', '''''','queueSize', [ 1;],'label', [ 0;],'ver', [ 2;],'showID', [ 0;],'showRaw', [ 0;],'showRawMsg', [ 0;],'showAge', [ 1;],'fill', [ 0;],'editID', [ 0;],'signalOrder', [ 1;],'signalAscDes', [ 1;])  canBus='CAN3'  mailbox=''  payloadMask=[]  payloadValue=[]  idMask=hex2dec('1FFFFFFF')  queueSize=1  showID=0  label=0  fill=0  id=1831  showRaw=0  showAge=1  signalOrder=1  signalInfo={{struct('Name', 'hbMC2','Startbit', [ 0;],'SignalSize', [ 8;],'ByteOrder', 'LittleEndian','ValueType', 'UNSIGNED','Class', 'uint8','Signed', [ 0;],'Factor', [ 1;],'Offset', [ 0;],'Min', [ 0;],'Max', [ 0;],'Units', '','Comment', '','StartBit', [ 0;])}}  showRawMsg=0
      settings: SourceProductName=Raptor
  raptor_can_rxmsg2 : Raptor_lib/CAN/raptor_can_rxmsg  canDefinition=struct('dbcFile', 'A1_MICH_EV_BOAT.dbc','message', 'heartBeatMC1','comment', '','signals', {{'hbMC1'}},'enabled', [ 1;],'scaled', [ 1;],'canBus', '''CAN3''','messageID', [ 1830;],'idMask', [ 536870911;],'payloadMask', [],'payloadValue', [],'period', [ 0;],'mailbox', '''''','queueSize', [ 1;],'label', [ 0;],'ver', [ 2;],'showID', [ 0;],'showRaw', [ 0;],'showRawMsg', [ 0;],'showAge', [ 1;],'fill', [ 0;],'editID', [ 0;],'signalOrder', [ 1;],'signalAscDes', [ 1;])  canBus='CAN3'  mailbox=''  payloadMask=[]  payloadValue=[]  idMask=hex2dec('1FFFFFFF')  queueSize=1  showID=0  label=0  fill=0  id=1830  showRaw=0  showAge=1  signalOrder=1  signalInfo={{struct('Name', 'hbMC1','Startbit', [ 0;],'SignalSize', [ 8;],'ByteOrder', 'LittleEndian','ValueType', 'UNSIGNED','Class', 'uint8','Signed', [ 0;],'Factor', [ 1;],'Offset', [ 0;],'Min', [ 0;],'Max', [ 0;],'Units', '','Comment', '','StartBit', [ 0;])}}  showRawMsg=0
      settings: SourceProductName=Raptor
  raptor_can_txmsg2 : Raptor_lib/CAN/raptor_can_txmsg  canDefinition=struct('dbcFile', 'A1_MICH_EV_BOAT.dbc','message', 'NMT','comment', '','signals', {{'id','o1'}},'enabled', [ 1 1;],'scaled', [ 1 1;],'canBus', '''CAN3''','messageID', [ 0;],'idMask', [ 536870911;],'payloadMask', [],'payloadValue', [],'period', [ 0;],'mailbox', '','queueSize', [ 1;],'label', [ 0;],'ver', [ 2;],'showID', [ 0;],'showRaw', [ 0;],'showRawMsg', [ 0;],'fill', [ 0;],'editID', [ 0;],'signalOrder', [ 1;],'signalAscDes', [ 1;])  canBus='CAN3'  queueSize=1  payloadMask=[]  payloadValue=[]  period=0  showID=0  label=0  idMask=hex2dec('1FFFFFFF')  fill=0  id=0  showRaw=0  signalOrder=1  signalInfo={{struct('Name', 'o1','Startbit', [ 0;],'SignalSize', [ 8;],'ByteOrder', 'LittleEndian','ValueType', 'UNSIGNED','Class', 'uint8','Signed', [ 0;],'Factor', [ 1;],'Offset', [ 0;],'Min', [ 0;],'Max', [ 0;],'Units', '','Comment', 'value 01 hex','StartBit', [ 0;]),struct('Name', 'id','Startbit', [ 0;],'SignalSize', [ 8;],'ByteOrder', 'LittleEndian','ValueType', 'UNSIGNED','Class', 'uint8','Signed', [ 0;],'Factor', [ 1;],'Offset', [ 0;],'Min', [ 0;],'Max', [ 0;],'Units', '','Comment', 'controller id hex (0x26 or 0x27 in our case)','StartBit', [ 8;])}}
      settings: SourceProductName=Raptor
  raptor_can_txmsg3 : Raptor_lib/CAN/raptor_can_txmsg  Commented=on  canDefinition=struct('dbcFile', 'A1_MICH_EV_BOAT.dbc','message', 'NMT','comment', '','signals', {{'id','o1'}},'enabled', [ 1 1;],'scaled', [ 1 1;],'canBus', '''CAN1''','messageID', [ 0;],'idMask', [ 536870911;],'payloadMask', [],'payloadValue', [],'period', [ 0;],'mailbox', '','queueSize', [ 1;],'label', [ 0;],'ver', [ 2;],'showID', [ 0;],'showRaw', [ 0;],'showRawMsg', [ 0;],'fill', [ 0;],'editID', [ 0;],'signalOrder', [ 1;],'signalAscDes', [ 1;])  canBus='CAN1'  queueSize=1  payloadMask=[]  payloadValue=[]  period=0  showID=0  label=0  idMask=hex2dec('1FFFFFFF')  fill=0  id=0  showRaw=0  signalOrder=1  signalInfo={{struct('Name', 'o1','Startbit', [ 0;],'SignalSize', [ 8;],'ByteOrder', 'LittleEndian','ValueType', 'UNSIGNED','Class', 'uint8','Signed', [ 0;],'Factor', [ 1;],'Offset', [ 0;],'Min', [ 0;],'Max', [ 0;],'Units', '','Comment', 'value 01 hex','StartBit', [ 0;]),struct('Name', 'id','Startbit', [ 0;],'SignalSize', [ 8;],'ByteOrder', 'LittleEndian','ValueType', 'UNSIGNED','Class', 'uint8','Signed', [ 0;],'Factor', [ 1;],'Offset', [ 0;],'Min', [ 0;],'Max', [ 0;],'Units', '','Comment', 'controller id hex (0x26 or 0x27 in our case)','StartBit', [ 8;])}}
      settings: SourceProductName=Raptor
  raptor_can_txmsg4 : Raptor_lib/CAN/raptor_can_txmsg  canDefinition=struct('dbcFile', 'A1_MICH_EV_BOAT.dbc','message', 'command1','comment', '','signals', {{'throttleCurrent1'}},'enabled', [ 1;],'scaled', [ 1;],'canBus', '''CAN3''','messageID', [ 550;],'idMask', [ 536870911;],'payloadMask', [],'payloadValue', [],'period', [ 0;],'mailbox', '','queueSize', [ 1;],'label', [ 0;],'ver', [ 2;],'showID', [ 0;],'showRaw', [ 0;],'showRawMsg', [ 0;],'fill', [ 0;],'editID', [ 0;],'signalOrder', [ 1;],'signalAscDes', [ 1;])  canBus='CAN3'  queueSize=1  payloadMask=[]  payloadValue=[]  period=0  showID=0  label=0  idMask=hex2dec('1FFFFFFF')  fill=0  id=550  showRaw=0  signalOrder=1  signalInfo={{struct('Name', 'throttleCurrent1','Startbit', [ 0;],'SignalSize', [ 16;],'ByteOrder', 'LittleEndian','ValueType', 'SIGNED','Class', 'int16','Signed', [ 1;],'Factor', [ 1;],'Offset', [ 0;],'Min', [ 0;],'Max', [ 0;],'Units', '','Comment', '','StartBit', [ 0;])}}
      settings: SourceProductName=Raptor
  raptor_can_txmsg5 : Raptor_lib/CAN/raptor_can_txmsg  canDefinition=struct('dbcFile', 'A1_MICH_EV_BOAT.dbc','message', 'command2','comment', '','signals', {{'throttleCurrent2'}},'enabled', [ 1;],'scaled', [ 1;],'canBus', '''CAN3''','messageID', [ 551;],'idMask', [ 536870911;],'payloadMask', [],'payloadValue', [],'period', [ 0;],'mailbox', '','queueSize', [ 1;],'label', [ 0;],'ver', [ 2;],'showID', [ 0;],'showRaw', [ 0;],'showRawMsg', [ 0;],'fill', [ 0;],'editID', [ 0;],'signalOrder', [ 1;],'signalAscDes', [ 1;])  canBus='CAN3'  queueSize=1  payloadMask=[]  payloadValue=[]  period=0  showID=0  label=0  idMask=hex2dec('1FFFFFFF')  fill=0  id=551  showRaw=0  signalOrder=1  signalInfo={{struct('Name', 'throttleCurrent2','Startbit', [ 0;],'SignalSize', [ 16;],'ByteOrder', 'LittleEndian','ValueType', 'SIGNED','Class', 'int16','Signed', [ 1;],'Factor', [ 1;],'Offset', [ 0;],'Min', [ 0;],'Max', [ 0;],'Units', '','Comment', '','StartBit', [ 0;])}}
      settings: SourceProductName=Raptor
  wires:
  RM/1 -> Product/1
  LM/1 -> Product1/1
  Product1/1 -> Gain/1
  If statement for on off switch2/1(Value out) -> Product1/2, Product/2
  Drive Mode/1 -> If statement for on off switch2/1(Switch Value)
  Gain/1 -> Saturation/1
  Motor Controller NMT id Switch/1(Value out) -> raptor_can_txmsg2/1
  Constant2/1 -> raptor_can_txmsg3/1
  Constant3/1 -> raptor_can_txmsg2/2
  Constant4/1 -> raptor_can_txmsg3/2
  Gain1/1 -> Saturation2/1
  raptor_can_rxmsg2/2 -> Motor Controller NMT id Switch/1(hbMC1)
  Product/1 -> Gain1/1
  Saturation2/1 -> Cast/1
  Cast/1 -> raptor_can_txmsg5/1
  Saturation/1 -> Cast1/1
  Cast1/1 -> raptor_can_txmsg4/1
  raptor_can_rxmsg1/2 -> Motor Controller NMT id Switch/2(hbMC2)

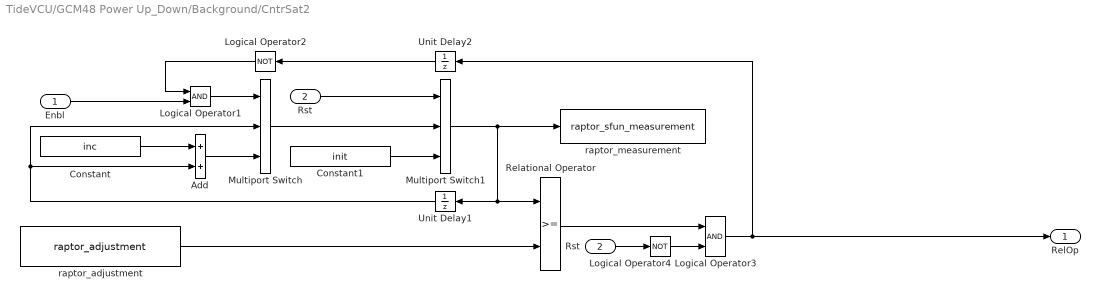
== system TideVCU/GCM48 Power Up_Down/Background/CntrSat2 ==
  Enbl : Inport
  Rst : Inport  Port=2
  Add : Sum  InputSameDT=on  OutDataTypeStr=Inherit: Same as first input
  Constant : Constant  Value=inc  OutDataTypeStr=uint32
  Constant1 : Constant  Value=init  OutDataTypeStr=uint32
  Logical Operator1 : Logic  OutDataTypeStr=boolean
  Logical Operator2 : Logic  Operator=NOT  Inputs=1  OutDataTypeStr=boolean
  Logical Operator3 : Logic  OutDataTypeStr=boolean
  Logical Operator4 : Logic  Operator=NOT  Inputs=1  OutDataTypeStr=boolean
  Multiport Switch : MultiPortSwitch  DataPortOrder=Zero-based contiguous  Inputs=2  zeroidx=on  InputSameDT=on
  Multiport Switch1 : MultiPortSwitch  DataPortOrder=Zero-based contiguous  Inputs=2  zeroidx=on  InputSameDT=on
  Relational Operator : RelationalOperator  OutDataTypeStr=boolean  RndMeth=Nearest
  "Rst " : InportShadow  Port=2
  Unit Delay1 : UnitDelay  InitialCondition=init  SampleTime=-1  HasFrameUpgradeWarning=on
  Unit Delay2 : UnitDelay  InitialCondition=boolean(0)  SampleTime=-1  HasFrameUpgradeWarning=on
  raptor_adjustment : Raptor_lib/Data Storage/raptor_adjustment  paramName=th_nam  nameSource=Parameter  initValue=.1 / th_gain  dataType=uint32  storage=Calibration  calDispType=Number  calEnum={'Disabled', 'Enabled'}  calGain=th_gain  calOffset=0  calMax=inf  calMin=-inf  calFormat='0.3'  calUnit=th_units  calHelp=th_help  calAccess=4  calFunction=th_group  calDispHeaders=off  calColHeaders={'Col1' 'Col2' 'Col3'}  calRowHeaders={'Row1' 'Row2' 'Row3'}
      settings: SourceProductName=Raptor
  raptor_measurement : S-Function  FunctionName=raptor_sfun_measurement  Parameters=char({dataName,''}), uint8(calDispType), char(enumName), int32(enumValue), double(calGain), double(calOffset), double(calMax), double(calMin), char(calUnit), char(calHelp), char(calFormat), char(calFunction), char(calAccess)  SFunctionDeploymentMode=off  EnableBusSupport=off  mask(Measurement){paramName=[th_nam(1:end-3) 'Tmr'], nameSource=Parameter, calDispType=Number, calEnum={'False', 'True'}, calGain=th_gain, calOffset=0.0, calMax=inf, calMin=-inf, calFormat='0.3', calUnit=th_units, calHelp=['time that gets compared to ' th_nam], calAccess=4, calFunction=th_group, calVisible=on}
      mask prompts: paramName "Name"; nameSource "Name Source"; calDispType "Display as"; calEnum "Enumeration Definition"; calGain "Gain"; calOffset "Offset"; calMax "Max"; calMin "Min"; calFormat "Display Decimal Places"; calUnit "Unit Text"; calHelp "Help Text"; calAccess "Access Level"; calFunction "Function"; calVisible "Visible in Cal"
      mask help: This block is used to display a value in the calibration tool.
      mask init:
      | raptor_sfun_measurement_maskInit;
      settings: MoveFcn=raptor_icon_redraw(gcb);
      mask Help: eval('raptor_help(''raptor_measurement'');')
      mask TypeOptions nameSource: Parameter | Input Wire
      mask Callback nameSource: raptor_sfun_measurement_dlgCb(gcb, 'nameSource');
      mask TypeOptions calDispType: Number | Enumeration | String
      mask Callback calDispType: raptor_sfun_measurement_dlgCb(gcb, 'calDispType');
      mask TypeOptions calAccess: 4 | 3 | 2 | 1
      mask Display: raptor_sfun_measurement_icon;
  RelOp : Outport  VectorParamsAs1DForOutWhenUnconnected=off
  wires:
  "Rst "/1 -> Logical Operator4/1
  Logical Operator4/1 -> Logical Operator3/2
  Relational Operator/1 -> Logical Operator3/1
  Multiport Switch1/1 -> Relational Operator/1, Unit Delay1/1, raptor_measurement/1
  Logical Operator2/1 -> Logical Operator1/1
  Constant1/1 -> Multiport Switch1/3
  Multiport Switch/1 -> Multiport Switch1/2
  Constant/1 -> Add/1
  Unit Delay1/1 -> Multiport Switch/2, Add/2
  Add/1 -> Multiport Switch/3
  Logical Operator1/1 -> Multiport Switch/1
  Enbl/1 -> Logical Operator1/2
  raptor_adjustment/1 -> Relational Operator/2
  Logical Operator3/1 -> RelOp/1, Unit Delay2/1
  Rst/1 -> Multiport Switch1/1
  Unit Delay2/1 -> Logical Operator2/1

== system TideVCU/GCM48 Power Up_Down/Background/Raise Shutdown Event ==
  init state = 1 to trigger at wakeup if awoken by a wake source that we want to ignore : TriggerPort  TriggerType=falling  VariantControl=Variant  InitialTriggerSignalState=positive
  Constant : Constant  Value=boolean(1)
  Function-Call Generator : simulink/Ports & Subsystems/Function-Call Generator  sample_time=-1  numberOfIterations=1  DisallowWideOutput=off
  raptor_data_def : Raptor_lib/Data Storage/raptor_data_def  dataName='FgndTasksStopped'  initValue=0  dataType=boolean  storage=Volatile (RAM)  calVisible=on  calType=Measurement  calDispType=Number  calEnum={'False', 'True'}  calGain=1.0  calOffset=0  calMin=-Inf  calMax=Inf  calFormat='-1'  calUnit='Bool'  calHelp='Boolean indicating foreground tasks stopped'  calAccess=4  calFunction=group  calDispHeaders=off  calColHeaders={'Col1' 'Col2' 'Col3'}  calRowHeaders={'Row1' 'Row2' 'Row3'}
      settings: SourceProductName=Raptor
  raptor_data_write : Raptor_lib/Data Storage/raptor_data_write  dataName='FgndTasksStopped'  dataShape=Scalar  idxSource=Input Port  idxRow=1  idxCol=1
      settings: SourceProductName=Raptor
  raptor_shutdown : Raptor_lib/Triggers/raptor_shutdown  null=0
      settings: SourceProductName=Raptor
  wires:
  Function-Call Generator/1 -> raptor_shutdown/Trigger
  Constant/1 -> raptor_data_write/1

== system TideVCU/GCM48 Power Up_Down/Background/Raise Startup Event ==
  note: - The Startup Event clears the flag "app_is_in_shutdown" in the c-code. Because this RAM flag initializes to zero anyway at startup, calling it here again is redundant. But leave it for clarity to the user.
      |
      | Also, this is NOT redundant in the case where the key turns back on during a shutdown. in that case, you definitely need this here
  init state zero so it triggers at wake if wake request is true : TriggerPort  VariantControl=Variant  InitialTriggerSignalState=zero  PortDimensions=1
  Constant : Constant  Value=boolean(1)
  Constant1 : Constant  Value=boolean(0)
  Function-Call Generator : simulink/Ports & Subsystems/Function-Call Generator  sample_time=-1  numberOfIterations=1  DisallowWideOutput=off
  raptor_data_write : Raptor_lib/Data Storage/raptor_data_write  dataName='FgndTasksStopped'  dataShape=Scalar  idxSource=Input Port  idxRow=1  idxCol=1
      settings: SourceProductName=Raptor
  raptor_measurement1 : Raptor_lib/Data Storage/raptor_measurement  paramName='Wake_Debug_StartupEventRaised'  nameSource=Parameter  calDispType=Number  calEnum={'False', 'True'}  calGain=1.0  calOffset=0.0  calMax=inf  calMin=-inf  calFormat='-1'  calUnit=''  calHelp=''  calAccess=4  calFunction=group  calVisible=on
      settings: SourceProductName=Raptor
  raptor_startup : Raptor_lib/Triggers/raptor_startup  null=0
      settings: SourceProductName=Raptor
  wires:
  Constant1/1 -> raptor_data_write/1
  Constant/1 -> raptor_measurement1/1
  Function-Call Generator/1 -> raptor_startup/Trigger

== system TideVCU/GCM48 Power Up_Down/Background/SR ==
  Set : Inport
  Rst : Inport  Port=2
  Constant : Constant  Value=boolean(0)
  Constant1 : Constant  Value=boolean(1)
  Multiport Switch : MultiPortSwitch  DataPortOrder=Zero-based contiguous  Inputs=2  zeroidx=on
  Multiport Switch1 : MultiPortSwitch  DataPortOrder=Zero-based contiguous  Inputs=2  zeroidx=on
  Unit Delay : UnitDelay  InitialCondition=init  SampleTime=-1  HasFrameUpgradeWarning=on
  Bool : Outport  VectorParamsAs1DForOutWhenUnconnected=off
  wires:
  Multiport Switch1/1 -> Multiport Switch/2
  Constant1/1 -> Multiport Switch1/3
  Constant/1 -> Multiport Switch/3
  Rst/1 -> Multiport Switch/1
  Set/1 -> Multiport Switch1/1
  Multiport Switch/1 -> Bool/1, Unit Delay/1
  Unit Delay/1 -> Multiport Switch1/2

== system TideVCU/GCM48 Power Up_Down/Background/Store EEPROM ==
  Trigger : TriggerPort  TriggerType=falling  VariantControl=Variant
  Function-Call Generator : simulink/Ports & Subsystems/Function-Call Generator  sample_time=-1  numberOfIterations=1  DisallowWideOutput=off
  raptor_store_nv : Raptor_lib/Data Storage/raptor_store_nv  null=0
      settings: SourceProductName=Raptor
  wires:
  Function-Call Generator/1 -> raptor_store_nv/Trigger
